simulink model "integrate_gyro"  (R2024b)
settings: Solver=FixedStepDiscrete  StartTime=t_0  StopTime=t_f  FixedStep=dt  RelTol=1e-8
undefined symbols (not defined in the file or in its folder): dt, ornt_init
libraries: sharedutil x1
settings Model: Creator=yevge  LastModifiedBy=Yevgeniy Gorbachev
settings DebuggingCC: AlgebraicLoopMsg=error  CheckMatrixSingularityMsg=error

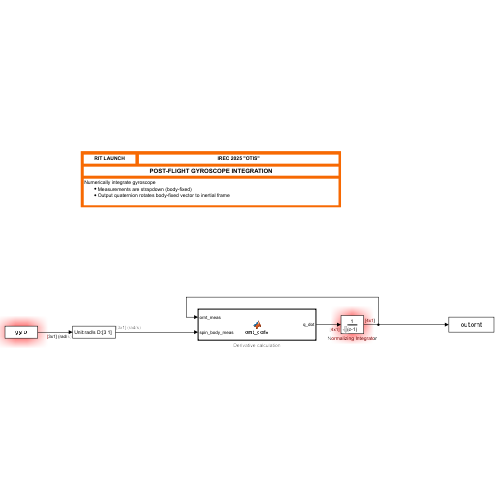
[thumbnail: Simulink's stored preview of the top-level diagram]
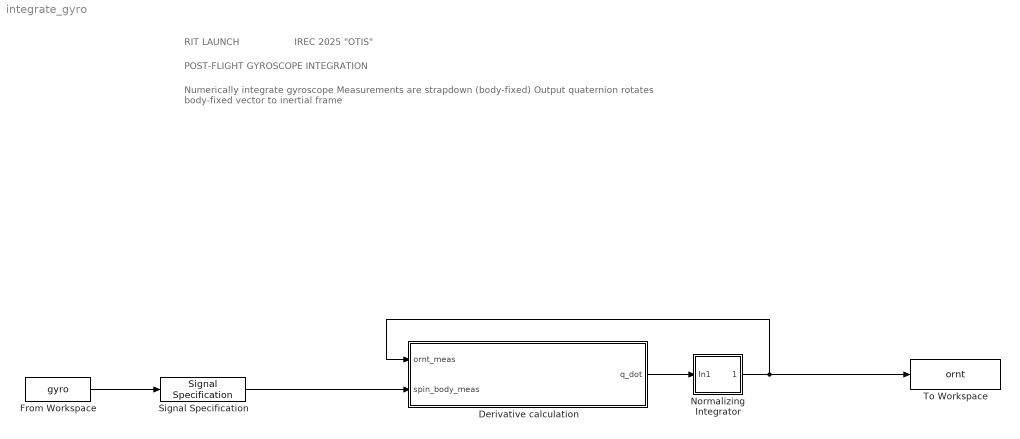
== system integrate_gyro ==
  note: POST-FLIGHT GYROSCOPE INTEGRATION
  note: IREC 2025 "OTIS"
  note: RIT LAUNCH
  note: Numerically integrate gyroscope
      | Measurements are strapdown (body-fixed)
      | Output quaternion rotates body-fixed vector to inertial frame
  Derivative calculation : MATLAB Function  TreatAsAtomicUnit=on
  From Workspace : FromWorkspace  VariableName=gyro  SampleTime=dt
  Normalizing Integrator : Subsystem  mask{T_s=dt, ornt_init=ornt_init}
      mask prompts: T_s "Sample time"; ornt_init "Initial orientation"
      mask Display: droots([], 1, '1', 'z');
  Signal Specification : SignalSpecification  Unit=rad/s  Dimensions=[3 1]
  To Workspace : ToWorkspace  VariableName=ornt  SaveFormat=Timeseries  SampleTime=-1
  wires:
  From Workspace/1 -> Signal Specification/1
  Normalizing Integrator/1(Out1) -> To Workspace/1, Derivative calculation/1(ornt_meas)
  Derivative calculation/1(q_dot) -> Normalizing Integrator/1(In1)
  Signal Specification/1 -> Derivative calculation/2(spin_body_meas)

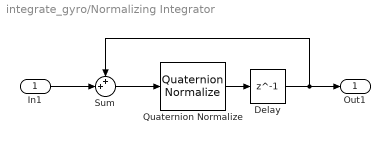
== system integrate_gyro/Normalizing Integrator ==
  In1 : Inport  PortDimensions=[4 1]
  Delay : Delay  DelayLength=1  InitialCondition=ornt_init
  Quaternion Normalize : sharedutil/Quaternion Normalize  aMode=aMode
  Sum : Sum  Inputs=++|
  Out1 : Outport  PortDimensions=[4 1]
  wires:
  In1/1 -> Sum/2
  Quaternion Normalize/1 -> Delay/1
  Sum/1 -> Quaternion Normalize/1
  Delay/1 -> Out1/1, Sum/1

== matlab function integrate_gyro/Derivative calculation ==
  data: ornt_meas input; q_dot output; spin_body_meas input
function q_dot = ornt_deriv(ornt_meas, spin_body_meas)
    q_dot = 0.5 .* quatmultiply(ornt_meas.', [0 spin_body_meas.']).';
end
